simulink model "Requriment_22"  (R2021a)
settings: Solver=FixedStepDiscrete  StartTime=0.0  StopTime=50  FixedStep=1  RelTol=1e-3
undefined symbols (not defined in the file): green_blink, green_on, red_blink, white_on, yellow_blink
libraries: simulink x7
settings Model: DataDictionary=charging_indicator_dd.sldd  EnableAccessToBaseWorkspace=off  Creator=Rahul  LastModifiedBy=Rahul

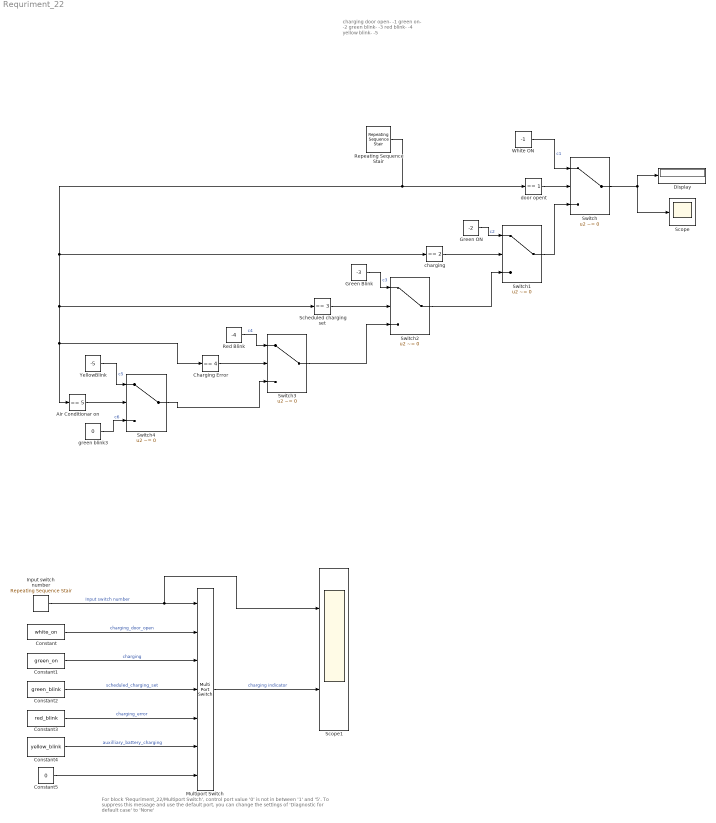
== system Requriment_22 ==
  note: For block 'Requriment_22/Multiport Switch', control port value '0' is not in between '1' and '5'. To suppress this message and use the default port, you can change the settings of 'Diagnostic for default case' to 'None'
  note: charging door open- -1
      | green on- -2
      | green blink-  -3
      | red blink- -4
      | yellow blink- -5
  "Air Conditionar on " : simulink/Logic and Bit Operations/Compare To Constant  relop===  const=5  OutDataTypeStr=boolean
  Charging Error : simulink/Logic and Bit Operations/Compare To Constant  relop===  const=4  OutDataTypeStr=boolean
  Constant : Constant  Value=white_on
  Constant1 : Constant  Value=green_on
  Constant2 : Constant  Value=green_blink
  Constant3 : Constant  Value=red_blink
  Constant4 : Constant  Value=yellow_blink
  Constant5 : Constant  Value=0
  Display : Display
  Green Blink : Constant  Value=-3
  Green ON : Constant  Value=-2
  Input switch number : simulink/Sources/Repeating Sequence Stair  OutValues=[3 5 8 2 9 1 0 4]  tsamp=-1  OutMin=[]  OutMax=[]  OutDataTypeStr=double  OutputDataTypeScalingMode=double  OutDataType=fixdt(0,8)  ConRadixGroup=Best Precision: Vector-wise  OutScaling=2^-12
  Multiport Switch : MultiPortSwitch  Inputs=5  DataPortForDefault=Additional data port  DiagnosticForDefault=Warning
  Red Blink : Constant  Value=-4
  Repeating Sequence Stair : simulink/Sources/Repeating Sequence Stair  OutValues="[0 1 3 11  5 0 3 2 5 1 4 1 3 5]"  tsamp=-1  OutMin=[]  OutMax=[]  OutDataTypeStr=double  OutputDataTypeScalingMode=double  OutDataType=fixdt(0,8)  ConRadixGroup=Best Precision: Vector-wise  OutScaling=2^-12
  "Scheduled charging set " : simulink/Logic and Bit Operations/Compare To Constant  relop===  const=3  OutDataTypeStr=boolean
  Scope : Scope
  Scope1 : Scope  NumInputPorts=2
  Switch{,1..4} (5 alike) : Switch  Criteria=u2 ~= 0
  White ON : Constant  Value=-1
  YellowBlink : Constant  Value=-5
  charging : simulink/Logic and Bit Operations/Compare To Constant  relop===  const=2  OutDataTypeStr=boolean
  door opent : simulink/Logic and Bit Operations/Compare To Constant  relop===  const=1  OutDataTypeStr=boolean
  green blink3 : Constant  Value=0
  wires:
  Switch1/1 -> Switch/3
  "Air Conditionar on "/1 -> Switch4/2
  "Scheduled charging set "/1 -> Switch2/2
  Switch4/1 -> Switch3/3
  Red Blink/1 -> Switch3/1  "c4"
  green blink3/1 -> Switch4/3  "c6"
  YellowBlink/1 -> Switch4/1  "c5"
  Green Blink/1 -> Switch2/1  "c3"
  Green ON/1 -> Switch1/1  "c2"
  charging/1 -> Switch1/2
  door opent/1 -> Switch/2
  Switch3/1 -> Switch2/3
  Switch/1 -> Display/1, Scope/1
  Switch2/1 -> Switch1/3
  Charging Error/1 -> Switch3/2
  Repeating Sequence Stair/1 -> "Air Conditionar on "/1, Charging Error/1, "Scheduled charging set "/1, charging/1, door opent/1
  White ON/1 -> Switch/1  "c1"
  Constant3/1 -> Multiport Switch/5  "charging_error"
  Constant4/1 -> Multiport Switch/6  "auxilliary_battery_charging"
  Constant/1 -> Multiport Switch/2  "charging_door_open"
  Constant1/1 -> Multiport Switch/3  "charging"
  Constant2/1 -> Multiport Switch/4  "scheduled_charging_set"
  Input switch number/1 -> Scope1/1, Multiport Switch/1  "Input switch number"
  Constant5/1 -> Multiport Switch/7
  Multiport Switch/1 -> Scope1/2  "charging indicator"
